simulink model "PID_controller"  (R2024a)
settings: Solver=VariableStepAuto  StartTime=0.0  StopTime=30  RelTol=1e-3
undefined symbols (not defined in the file): KD, KI, KP
libraries: simulink x1
settings Model: Creator=tinas  LastModifiedBy=umara

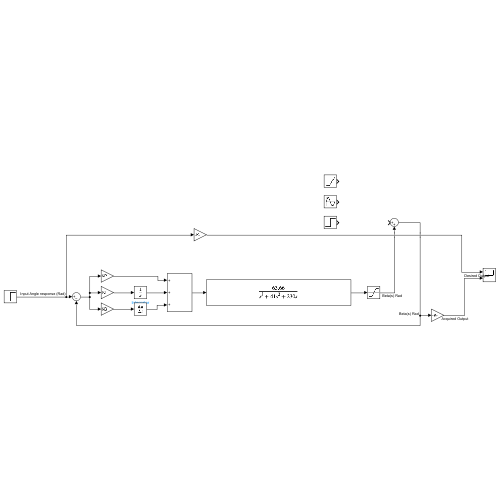
[thumbnail: Simulink's stored preview of the top-level diagram]
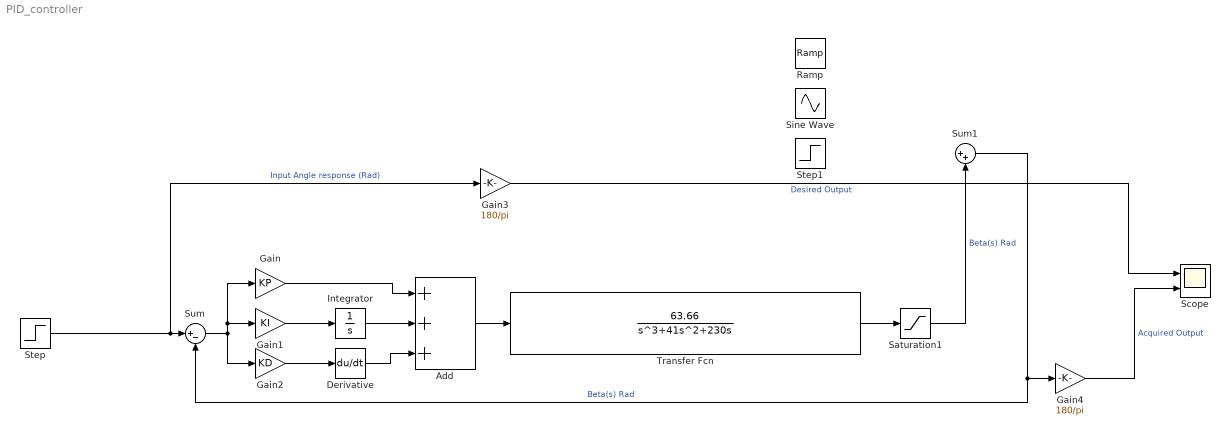
== system PID_controller ==
  Add : Sum  Inputs=+++
  Derivative : Derivative
  Gain : Gain  Gain=KP
  Gain1 : Gain  Gain=KI
  Gain2 : Gain  Gain=KD
  Gain3 : Gain  Gain=180/pi
  Gain4 : Gain  Gain=180/pi
  Integrator : Integrator
  Ramp : simulink/Sources/Ramp  slope=(90)/(12*3600)  start=0  InitialOutput=0
  Saturation1 : Saturate  UpperLimit=135*pi/180  LowerLimit=-pi/2
  Scope : Scope  NumInputPorts=2
  Sine Wave : Sin  Amplitude=15*pi/180  SampleTime=0
  Step : Step  Time=0  After=45*pi/180  SampleTime=0
  Step1 : Step  Time=10  After=45*pi/180  SampleTime=0
  Sum : Sum  Inputs=|+-
  Sum1 : Sum  Inputs=|++
  Transfer Fcn : TransferFcn  Numerator=[63.66]  Denominator="[1   41  230  0]"
  wires:
  Add/1 -> Transfer Fcn/1
  Gain/1 -> Add/1
  Integrator/1 -> Add/2
  Gain1/1 -> Integrator/1
  Derivative/1 -> Add/3
  Gain2/1 -> Derivative/1
  Step/1 -> Gain3/1, Sum/1  "Input Angle response (Rad)"
  Sum/1 -> Gain/1, Gain1/1, Gain2/1
  Transfer Fcn/1 -> Saturation1/1
  Sum1/1 -> Gain4/1, Sum/2  "Beta(s) Rad"
  Gain3/1 -> Scope/1  "Desired Output"
  Gain4/1 -> Scope/2  "Acquired Output"
  Saturation1/1 -> Sum1/2  "Beta(s) Rad"
